simulink model "controller"  (R2024b)
settings: Solver=FixedStepDiscrete  StartTime=0.0  StopTime=30  FixedStep=0.01  RelTol=1e-3
model workspace (MAT data in the model file):
  roll = 1
undefined symbols (not defined in the file or in its folder): f
libraries: eeGeneralControl x12, slpidlib x8, dspstat3 x4, instrumentlib x4
settings Model: Creator=PC  LastModifiedBy=PC

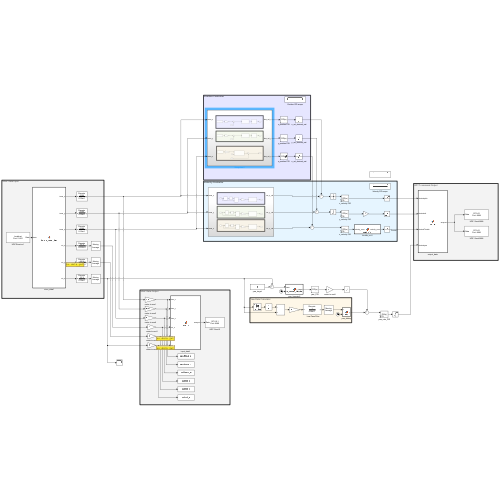
[thumbnail: Simulink's stored preview of the top-level diagram]
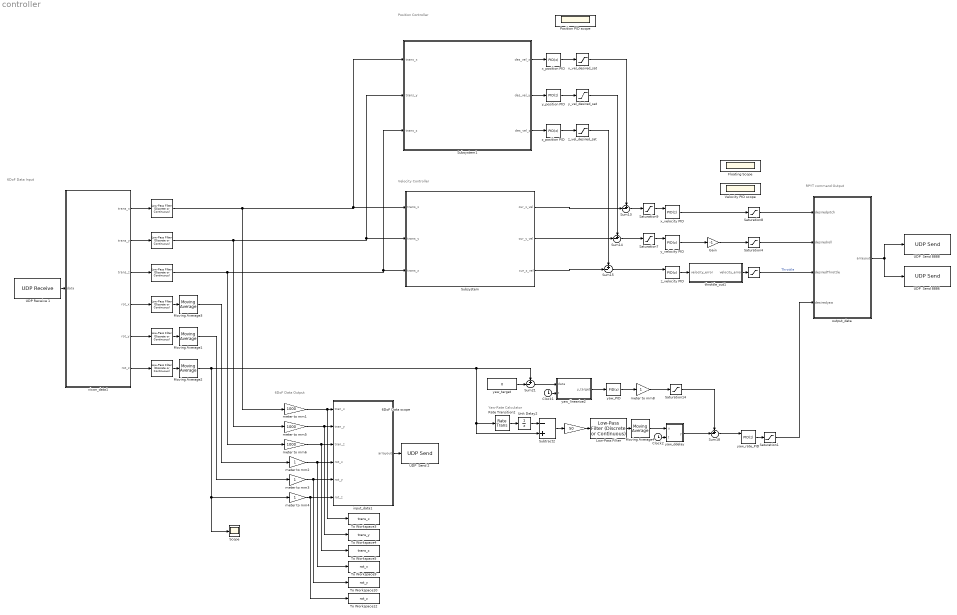
== system controller ==
  note: Velocity Controller
  note: Position Controller
  note: Yaw-Rate Calculator
  note: 6DoF Data Output
  note: 6DoF Data Input
  note: RPYT command Output
  "   " : Saturate  UpperLimit=20000  LowerLimit=0
  "    " : eeGeneralControl/Low-Pass Filter (Discrete or Continuous)  K=0.001  T=0.03  B=inf  A=-inf  init_option=Inherited from block input  x0=0  Ts=0.01
  "               " : Gain  Gain=50
  "                                       " : eeGeneralControl/Low-Pass Filter (Discrete or Continuous)  K=0.001  T=0.03  B=inf  A=-inf  init_option=Inherited from block input  x0=0  Ts=0.01
  "                                                    " : eeGeneralControl/Low-Pass Filter (Discrete or Continuous)  K=57.3  T=0.016  B=inf  A=-inf  init_option=Inherited from block input  x0=0  Ts=0.01
  "                                                      " : eeGeneralControl/Low-Pass Filter (Discrete or Continuous)  K=57.3  T=0.016  B=inf  A=-inf  init_option=Inherited from block input  x0=0  Ts=0.01
  "                                                           " : eeGeneralControl/Low-Pass Filter (Discrete or Continuous)  K=0.001  T=0.03  B=inf  A=-inf  init_option=Inherited from block input  x0=0  Ts=0.01
  "                                                                                           " : eeGeneralControl/Low-Pass Filter (Discrete or Continuous)  K=57.3  T=0.03  B=inf  A=-inf  init_option=Inherited from block input  x0=0  Ts=0.01
  "    Low-Pass Filter" : eeGeneralControl/Low-Pass Filter (Discrete or Continuous)  K=1  T=0.08  B=inf  A=-inf  init_option=Inherited from block input  x0=0  Ts=0.01
  6DoF Data scope : Scope
      settings: Floating=on
  Clock1 : Clock
  Clock2 : Clock
  Floating Scope : Scope
      settings: Floating=on
  Gain : Gain  Gain=-1
  Moving Average1 : dspstat3/Moving Average  Method=Sliding window  ForgettingFactorPort=off  SpecifyWindowLength=on  WindowLength=8  OverlapLength=7  AllowArbitraryInputLength=off  ForgettingFactor=0.9  SimulateUsing=Interpreted execution
  Moving Average2 : dspstat3/Moving Average  Method=Sliding window  ForgettingFactorPort=off  SpecifyWindowLength=on  WindowLength=15  OverlapLength=14  AllowArbitraryInputLength=off  ForgettingFactor=0.9  SimulateUsing=Interpreted execution
  Moving Average3 : dspstat3/Moving Average  Method=Sliding window  ForgettingFactorPort=off  SpecifyWindowLength=on  WindowLength=8  OverlapLength=7  AllowArbitraryInputLength=off  ForgettingFactor=0.9  SimulateUsing=Interpreted execution
  Moving Average4 : dspstat3/Moving Average  Method=Sliding window  ForgettingFactorPort=off  SpecifyWindowLength=on  WindowLength=30  OverlapLength=29  AllowArbitraryInputLength=off  ForgettingFactor=0.9  SimulateUsing=Interpreted execution
  Position PID scope : Scope
      settings: Floating=on
  Rate Transition2 : RateTransition  OutPortSampleTime=0.02
  Saturation1 : Saturate  UpperLimit=10  LowerLimit=-10
  Saturation14 : Saturate  UpperLimit=25  LowerLimit=-25
  Saturation4 : Saturate  UpperLimit=5  LowerLimit=-5
  Saturation7 : Saturate  UpperLimit=0.8  LowerLimit=-0.8
  Saturation8 : Saturate  UpperLimit=5  LowerLimit=-5
  Saturation9 : Saturate  UpperLimit=0.8  LowerLimit=-0.8
  Scope : Scope
  Subsystem : Subsystem
  Subsystem1 : Subsystem
  Subtract2 : Sum  Inputs=-+
  Sum{13..15,18,21} (5 alike) : Sum  Inputs=+-|
  To Workspace10 : ToWorkspace  VariableName=rot_y  SaveFormat=Timeseries  SampleTime=-1
  To Workspace12 : ToWorkspace  VariableName=rot_z  SaveFormat=Timeseries  SampleTime=-1
  To Workspace3 : ToWorkspace  VariableName=trans_x  SaveFormat=Timeseries  SampleTime=-1
  To Workspace4 : ToWorkspace  VariableName=trans_y  SaveFormat=Timeseries  SampleTime=-1
  To Workspace5 : ToWorkspace  VariableName=trans_z  SaveFormat=Timeseries  SampleTime=-1
  To Workspace9 : ToWorkspace  VariableName=rot_x  SaveFormat=Timeseries  SampleTime=-1
  UDP  Send 2 : instrumentlib/UDP Send  Host=127.0.0.1  Port=8889  LocalAddress=0.0.0.0  LocalPort=-1  EnablePortSharing=off  OutputDatagramPacketSize=2048  ByteOrder=big-endian  EnableBlockingMode=on  SimulateUsing=Interpreted execution
  UDP  Send 8886 : instrumentlib/UDP Send  Host=127.0.0.1  Port=8886  LocalAddress=0.0.0.0  LocalPort=-1  EnablePortSharing=off  OutputDatagramPacketSize=2048  ByteOrder=big-endian  EnableBlockingMode=on  SimulateUsing=Interpreted execution
  UDP  Send 8888 : instrumentlib/UDP Send  Host=127.0.0.1  Port=8888  LocalAddress=0.0.0.0  LocalPort=-1  EnablePortSharing=off  OutputDatagramPacketSize=2048  ByteOrder=big-endian  EnableBlockingMode=on  SimulateUsing=Interpreted execution
  UDP Receive 1 : instrumentlib/UDP Receive  LocalAddress=localhost  LocalPort=51001  EnablePortSharing=on  Host=localhost  Port=9090  GetLatestData=on  DataSize=[1024, 1]  DataType=uint8  ASCIIFormatting=%f,  Terminator=LF  CustomTerminator=10  ByteOrder=big-endian  EnableBlockingMode=on  Timeout=5  SampleTime=0.01  SimulateUsing=Interpreted execution
  Unit Delay2 : UnitDelay  SampleTime=0.01  HasFrameUpgradeWarning=on
  Velocity PID scope : Scope
      settings: Floating=on
  input_data1 : MATLAB Function  TreatAsAtomicUnit=on
  meter to mm1 : Gain  Gain=1000
  meter to mm{2..4,8} (4 alike) : Gain
  meter to mm5 : Gain  Gain=1000
  meter to mm6 : Gain  Gain=1000
  output_data : MATLAB Function  TreatAsAtomicUnit=on
  throttle_out1 : MATLAB Function  TreatAsAtomicUnit=on
  vicon_data1 : MATLAB Function  TreatAsAtomicUnit=on
  x_position PID : slpidlib/PID Controller  Controller=PID  Form=Parallel  TimeDomain=Discrete-time  UseExternalTs=off  SampleTime=-1  IntegratorMethod=Forward Euler  FilterMethod=Forward Euler  ControllerParametersSource=internal  P=2  I=0.1  UseKiTs=off  D=0.7  UseExternalDerivativeSource=off  N=50  UseFilter=on  TunerSelectOption=Transfer Function Based (PID Tuner App)  InitialConditionSource=internal  InitialConditionForIntegrator=0  InitialConditionForFilter=0  DifferentiatorICPrevScaledInput=0  ExternalReset=none  TrackingMode=off  Kt=0.1  LimitOutput=off  SatLimitsSource=internal  UpperSaturationLimit=inf  LowerSaturationLimit=-inf  LinearizeAsGain=on  AntiWindupMode=none  Kb=1  LimitIntegrator=on  UpperIntegratorSaturationLimit=0.5  LowerIntegratorSaturationLimit=-0.5  POutMin=[]  POutMax=[]  IOutMin=[]  IOutMax=[]  DOutMin=[]  DOutMax=[]  NOutMin=[]  NOutMax=[]  SumOutMin=[]  SumOutMax=[]  SaturationOutMin=[]  SaturationOutMax=[]  PParamMin=[]  PParamMax=[]  IParamMin=[]  IParamMax=[]  DParamMin=[]  DParamMax=[]  NParamMin=[]  NParamMax=[]  KbParamMin=[]  KbParamMax=[]  KtParamMin=[]  KtParamMax=[]  KbOutMin=[]  KbOutMax=[]  KtOutMin=[]  KtOutMax=[]  IntegratorOutMin=[]  IntegratorOutMax=[]  FilterOutMin=[]  FilterOutMax=[]  SumI1OutMin=[]  SumI1OutMax=[]  SumI2OutMin=[]  SumI2OutMax=[]  SumI3OutMin=[]  SumI3OutMax=[]  SumI4OutMin=[]  SumI4OutMax=[]  SumDOutMin=[]  SumDOutMax=[]  DifferentiatorOutMin=[]  DifferentiatorOutMax=[]  FilterDiffOutCoefMin=[]  FilterDiffOutCoefMax=[]  ReciprocalOutMin=[]  ReciprocalOutMax=[]  SumDenOutMin=[]  SumDenOutMax=[]  SumNumOutMin=[]  SumNumOutMax=[]  DivideOutMin=[]  DivideOutMax=[]  UdiffTsProdOutMin=[]  UdiffTsProdOutMax=[]  NTsProdOutMin=[]  NTsProdOutMax=[]  UintegralTsProdOutMin=[]  UintegralTsProdOutMax=[]  UngainTsProdOutMin=[]  UngainTsProdOutMax=[]  ClampingZeroOutDataTypeStr=Inherit: Inherit via back propagation  ClampingZeroOutMin=[]  ClampingZeroOutMax=[]  FilterDenConstantOutDataTypeStr=Inherit: Inherit via back propagation  FilterDenConstantOutMin=[]  FilterDenConstantOutMax=[]  PCopyOutDataTypeStr=Inherit: Inherit via back propagation  PCopyOutMin=[]  PCopyOutMax=[]  NCopyOutDataTypeStr=Inherit: Inherit via back propagation  NCopyOutMin=[]  NCopyOutMax=[]  IntegratorContinuousStateAttributes=''  IntegratorStateMustResolveToSignalObject=off  IntegratorRTWStateStorageClass=Auto  FilterContinuousStateAttributes=''  FilterStateMustResolveToSignalObject=off  FilterRTWStateStorageClass=Auto  ParallelPVariant=InternalParameters  IdealPVariant=Disabled  IVariant=InternalParameters  DVariant=InternalParameters  IntegratorVariant=Discrete  SatVariant=Disabled  AWVariant=Passthrough  PCopyVariant=Disabled  TRVariant=Disabled  FdbkBlocksVariant=Forward  IdealPFdbkVariant=Disabled  SatFdbkVariant=Disabled  DerivativeFilterVariant=ForwardEulerFilter  NVariant=InternalParameters  NCopyVariant=Disabled  FilterICVariant=InternalICsFilter  IntegratorICVariant=InternalICs  ExternalResetVariant=Disabled  TRSumVariant=Passthrough  SumFdbkVariant=Disabled  SumVariant=Sum_PID  TsampFilterVariant=InternalTs  TsampNgainVariant=Passthrough  TsampIntegralVariant=Disabled_SignalSpec  ExternalSaturationOutDataTypeStr=Inherit: Same as second input  DerivativeSourceVariant=ErrorSignal  PreIntVariant=InternalPreInt
  x_vel_desired_sat : Saturate  UpperLimit=1.2  LowerLimit=-1.2
  x_velocity PID : slpidlib/PID Controller  Controller=PID  Form=Parallel  TimeDomain=Discrete-time  UseExternalTs=off  SampleTime=-1  IntegratorMethod=Forward Euler  FilterMethod=Forward Euler  ControllerParametersSource=internal  P=2  I=0.2  UseKiTs=off  D=0.4  UseExternalDerivativeSource=off  N=50  UseFilter=on  TunerSelectOption=Transfer Function Based (PID Tuner App)  InitialConditionSource=internal  InitialConditionForIntegrator=0  InitialConditionForFilter=0  DifferentiatorICPrevScaledInput=0  ExternalReset=none  TrackingMode=on  Kt=1.5  LimitOutput=off  SatLimitsSource=internal  UpperSaturationLimit=inf  LowerSaturationLimit=-inf  LinearizeAsGain=on  AntiWindupMode=none  Kb=1  LimitIntegrator=on  UpperIntegratorSaturationLimit=0.3  LowerIntegratorSaturationLimit=-0.3  POutMin=[]  POutMax=[]  IOutMin=[]  IOutMax=[]  DOutMin=[]  DOutMax=[]  NOutMin=[]  NOutMax=[]  SumOutMin=[]  SumOutMax=[]  SaturationOutMin=[]  SaturationOutMax=[]  PParamMin=[]  PParamMax=[]  IParamMin=[]  IParamMax=[]  DParamMin=[]  DParamMax=[]  NParamMin=[]  NParamMax=[]  KbParamMin=[]  KbParamMax=[]  KtParamMin=[]  KtParamMax=[]  KbOutMin=[]  KbOutMax=[]  KtOutMin=[]  KtOutMax=[]  IntegratorOutMin=[]  IntegratorOutMax=[]  FilterOutMin=[]  FilterOutMax=[]  SumI1OutMin=[]  SumI1OutMax=[]  SumI2OutMin=[]  SumI2OutMax=[]  SumI3OutMin=[]  SumI3OutMax=[]  SumI4OutMin=[]  SumI4OutMax=[]  SumDOutMin=[]  SumDOutMax=[]  DifferentiatorOutMin=[]  DifferentiatorOutMax=[]  FilterDiffOutCoefMin=[]  FilterDiffOutCoefMax=[]  ReciprocalOutMin=[]  ReciprocalOutMax=[]  SumDenOutMin=[]  SumDenOutMax=[]  SumNumOutMin=[]  SumNumOutMax=[]  DivideOutMin=[]  DivideOutMax=[]  UdiffTsProdOutMin=[]  UdiffTsProdOutMax=[]  NTsProdOutMin=[]  NTsProdOutMax=[]  UintegralTsProdOutMin=[]  UintegralTsProdOutMax=[]  UngainTsProdOutMin=[]  UngainTsProdOutMax=[]  ClampingZeroOutDataTypeStr=Inherit: Inherit via back propagation  ClampingZeroOutMin=[]  ClampingZeroOutMax=[]  FilterDenConstantOutDataTypeStr=Inherit: Inherit via back propagation  FilterDenConstantOutMin=[]  FilterDenConstantOutMax=[]  PCopyOutDataTypeStr=Inherit: Inherit via back propagation  PCopyOutMin=[]  PCopyOutMax=[]  NCopyOutDataTypeStr=Inherit: Inherit via back propagation  NCopyOutMin=[]  NCopyOutMax=[]  IntegratorContinuousStateAttributes=''  IntegratorStateMustResolveToSignalObject=off  IntegratorRTWStateStorageClass=Auto  FilterContinuousStateAttributes=''  FilterStateMustResolveToSignalObject=off  FilterRTWStateStorageClass=Auto  ParallelPVariant=InternalParameters  IdealPVariant=Disabled  IVariant=InternalParameters  DVariant=InternalParameters  IntegratorVariant=Discrete  SatVariant=Disabled  AWVariant=Passthrough  PCopyVariant=Disabled  TRVariant=Enabled  FdbkBlocksVariant=Forward  IdealPFdbkVariant=Disabled  SatFdbkVariant=Disabled  DerivativeFilterVariant=ForwardEulerFilter  NVariant=InternalParameters  NCopyVariant=Disabled  FilterICVariant=InternalICsFilter  IntegratorICVariant=InternalICs  ExternalResetVariant=Disabled  TRSumVariant=TrackingMode  SumFdbkVariant=Disabled  SumVariant=Sum_PID  TsampFilterVariant=InternalTs  TsampNgainVariant=Passthrough  TsampIntegralVariant=Disabled_SignalSpec  ExternalSaturationOutDataTypeStr=Inherit: Same as second input  DerivativeSourceVariant=ErrorSignal  PreIntVariant=InternalPreInt
  y_position PID : slpidlib/PID Controller  Controller=PID  Form=Parallel  TimeDomain=Discrete-time  UseExternalTs=off  SampleTime=-1  IntegratorMethod=Forward Euler  FilterMethod=Forward Euler  ControllerParametersSource=internal  P=2  I=0.1  UseKiTs=off  D=0.7  UseExternalDerivativeSource=off  N=50  UseFilter=on  TunerSelectOption=Transfer Function Based (PID Tuner App)  InitialConditionSource=internal  InitialConditionForIntegrator=0  InitialConditionForFilter=0  DifferentiatorICPrevScaledInput=0  ExternalReset=none  TrackingMode=off  Kt=0.1  LimitOutput=off  SatLimitsSource=internal  UpperSaturationLimit=inf  LowerSaturationLimit=-inf  LinearizeAsGain=on  AntiWindupMode=none  Kb=1  LimitIntegrator=on  UpperIntegratorSaturationLimit=0.5  LowerIntegratorSaturationLimit=-0.5  POutMin=[]  POutMax=[]  IOutMin=[]  IOutMax=[]  DOutMin=[]  DOutMax=[]  NOutMin=[]  NOutMax=[]  SumOutMin=[]  SumOutMax=[]  SaturationOutMin=[]  SaturationOutMax=[]  PParamMin=[]  PParamMax=[]  IParamMin=[]  IParamMax=[]  DParamMin=[]  DParamMax=[]  NParamMin=[]  NParamMax=[]  KbParamMin=[]  KbParamMax=[]  KtParamMin=[]  KtParamMax=[]  KbOutMin=[]  KbOutMax=[]  KtOutMin=[]  KtOutMax=[]  IntegratorOutMin=[]  IntegratorOutMax=[]  FilterOutMin=[]  FilterOutMax=[]  SumI1OutMin=[]  SumI1OutMax=[]  SumI2OutMin=[]  SumI2OutMax=[]  SumI3OutMin=[]  SumI3OutMax=[]  SumI4OutMin=[]  SumI4OutMax=[]  SumDOutMin=[]  SumDOutMax=[]  DifferentiatorOutMin=[]  DifferentiatorOutMax=[]  FilterDiffOutCoefMin=[]  FilterDiffOutCoefMax=[]  ReciprocalOutMin=[]  ReciprocalOutMax=[]  SumDenOutMin=[]  SumDenOutMax=[]  SumNumOutMin=[]  SumNumOutMax=[]  DivideOutMin=[]  DivideOutMax=[]  UdiffTsProdOutMin=[]  UdiffTsProdOutMax=[]  NTsProdOutMin=[]  NTsProdOutMax=[]  UintegralTsProdOutMin=[]  UintegralTsProdOutMax=[]  UngainTsProdOutMin=[]  UngainTsProdOutMax=[]  ClampingZeroOutDataTypeStr=Inherit: Inherit via back propagation  ClampingZeroOutMin=[]  ClampingZeroOutMax=[]  FilterDenConstantOutDataTypeStr=Inherit: Inherit via back propagation  FilterDenConstantOutMin=[]  FilterDenConstantOutMax=[]  PCopyOutDataTypeStr=Inherit: Inherit via back propagation  PCopyOutMin=[]  PCopyOutMax=[]  NCopyOutDataTypeStr=Inherit: Inherit via back propagation  NCopyOutMin=[]  NCopyOutMax=[]  IntegratorContinuousStateAttributes=''  IntegratorStateMustResolveToSignalObject=off  IntegratorRTWStateStorageClass=Auto  FilterContinuousStateAttributes=''  FilterStateMustResolveToSignalObject=off  FilterRTWStateStorageClass=Auto  ParallelPVariant=InternalParameters  IdealPVariant=Disabled  IVariant=InternalParameters  DVariant=InternalParameters  IntegratorVariant=Discrete  SatVariant=Disabled  AWVariant=Passthrough  PCopyVariant=Disabled  TRVariant=Disabled  FdbkBlocksVariant=Forward  IdealPFdbkVariant=Disabled  SatFdbkVariant=Disabled  DerivativeFilterVariant=ForwardEulerFilter  NVariant=InternalParameters  NCopyVariant=Disabled  FilterICVariant=InternalICsFilter  IntegratorICVariant=InternalICs  ExternalResetVariant=Disabled  TRSumVariant=Passthrough  SumFdbkVariant=Disabled  SumVariant=Sum_PID  TsampFilterVariant=InternalTs  TsampNgainVariant=Passthrough  TsampIntegralVariant=Disabled_SignalSpec  ExternalSaturationOutDataTypeStr=Inherit: Same as second input  DerivativeSourceVariant=ErrorSignal  PreIntVariant=InternalPreInt
  y_vel_desired_sat : Saturate  UpperLimit=1.2  LowerLimit=-1.2
  y_velocity PID : slpidlib/PID Controller  Controller=PID  Form=Parallel  TimeDomain=Discrete-time  UseExternalTs=off  SampleTime=-1  IntegratorMethod=Forward Euler  FilterMethod=Forward Euler  ControllerParametersSource=internal  P=3.2  I=0.06  UseKiTs=off  D=0.25  UseExternalDerivativeSource=off  N=50  UseFilter=on  TunerSelectOption=Transfer Function Based (PID Tuner App)  InitialConditionSource=internal  InitialConditionForIntegrator=0  InitialConditionForFilter=0  DifferentiatorICPrevScaledInput=0  ExternalReset=none  TrackingMode=on  Kt=1.7  LimitOutput=off  SatLimitsSource=internal  UpperSaturationLimit=inf  LowerSaturationLimit=-inf  LinearizeAsGain=on  AntiWindupMode=none  Kb=1  LimitIntegrator=on  UpperIntegratorSaturationLimit=0.3  LowerIntegratorSaturationLimit=-0.3  POutMin=[]  POutMax=[]  IOutMin=[]  IOutMax=[]  DOutMin=[]  DOutMax=[]  NOutMin=[]  NOutMax=[]  SumOutMin=[]  SumOutMax=[]  SaturationOutMin=[]  SaturationOutMax=[]  PParamMin=[]  PParamMax=[]  IParamMin=[]  IParamMax=[]  DParamMin=[]  DParamMax=[]  NParamMin=[]  NParamMax=[]  KbParamMin=[]  KbParamMax=[]  KtParamMin=[]  KtParamMax=[]  KbOutMin=[]  KbOutMax=[]  KtOutMin=[]  KtOutMax=[]  IntegratorOutMin=[]  IntegratorOutMax=[]  FilterOutMin=[]  FilterOutMax=[]  SumI1OutMin=[]  SumI1OutMax=[]  SumI2OutMin=[]  SumI2OutMax=[]  SumI3OutMin=[]  SumI3OutMax=[]  SumI4OutMin=[]  SumI4OutMax=[]  SumDOutMin=[]  SumDOutMax=[]  DifferentiatorOutMin=[]  DifferentiatorOutMax=[]  FilterDiffOutCoefMin=[]  FilterDiffOutCoefMax=[]  ReciprocalOutMin=[]  ReciprocalOutMax=[]  SumDenOutMin=[]  SumDenOutMax=[]  SumNumOutMin=[]  SumNumOutMax=[]  DivideOutMin=[]  DivideOutMax=[]  UdiffTsProdOutMin=[]  UdiffTsProdOutMax=[]  NTsProdOutMin=[]  NTsProdOutMax=[]  UintegralTsProdOutMin=[]  UintegralTsProdOutMax=[]  UngainTsProdOutMin=[]  UngainTsProdOutMax=[]  ClampingZeroOutDataTypeStr=Inherit: Inherit via back propagation  ClampingZeroOutMin=[]  ClampingZeroOutMax=[]  FilterDenConstantOutDataTypeStr=Inherit: Inherit via back propagation  FilterDenConstantOutMin=[]  FilterDenConstantOutMax=[]  PCopyOutDataTypeStr=Inherit: Inherit via back propagation  PCopyOutMin=[]  PCopyOutMax=[]  NCopyOutDataTypeStr=Inherit: Inherit via back propagation  NCopyOutMin=[]  NCopyOutMax=[]  IntegratorContinuousStateAttributes=''  IntegratorStateMustResolveToSignalObject=off  IntegratorRTWStateStorageClass=Auto  FilterContinuousStateAttributes=''  FilterStateMustResolveToSignalObject=off  FilterRTWStateStorageClass=Auto  ParallelPVariant=InternalParameters  IdealPVariant=Disabled  IVariant=InternalParameters  DVariant=InternalParameters  IntegratorVariant=Discrete  SatVariant=Disabled  AWVariant=Passthrough  PCopyVariant=Disabled  TRVariant=Enabled  FdbkBlocksVariant=Forward  IdealPFdbkVariant=Disabled  SatFdbkVariant=Disabled  DerivativeFilterVariant=ForwardEulerFilter  NVariant=InternalParameters  NCopyVariant=Disabled  FilterICVariant=InternalICsFilter  IntegratorICVariant=InternalICs  ExternalResetVariant=Disabled  TRSumVariant=TrackingMode  SumFdbkVariant=Disabled  SumVariant=Sum_PID  TsampFilterVariant=InternalTs  TsampNgainVariant=Passthrough  TsampIntegralVariant=Disabled_SignalSpec  ExternalSaturationOutDataTypeStr=Inherit: Same as second input  DerivativeSourceVariant=ErrorSignal  PreIntVariant=InternalPreInt
  yaw_PID : slpidlib/PID Controller  Controller=PID  Form=Parallel  TimeDomain=Discrete-time  UseExternalTs=off  SampleTime=-1  IntegratorMethod=Forward Euler  FilterMethod=Forward Euler  ControllerParametersSource=internal  P=0.3  I=0.05  UseKiTs=off  D=0  UseExternalDerivativeSource=off  N=50  UseFilter=on  TunerSelectOption=Transfer Function Based (PID Tuner App)  InitialConditionSource=internal  InitialConditionForIntegrator=0  InitialConditionForFilter=0  DifferentiatorICPrevScaledInput=0  ExternalReset=none  TrackingMode=off  Kt=4  LimitOutput=off  SatLimitsSource=internal  UpperSaturationLimit=inf  LowerSaturationLimit=-inf  LinearizeAsGain=on  AntiWindupMode=none  Kb=1  LimitIntegrator=on  UpperIntegratorSaturationLimit=2  LowerIntegratorSaturationLimit=-2  POutMin=[]  POutMax=[]  IOutMin=[]  IOutMax=[]  DOutMin=[]  DOutMax=[]  NOutMin=[]  NOutMax=[]  SumOutMin=[]  SumOutMax=[]  SaturationOutMin=[]  SaturationOutMax=[]  PParamMin=[]  PParamMax=[]  IParamMin=[]  IParamMax=[]  DParamMin=[]  DParamMax=[]  NParamMin=[]  NParamMax=[]  KbParamMin=[]  KbParamMax=[]  KtParamMin=[]  KtParamMax=[]  KbOutMin=[]  KbOutMax=[]  KtOutMin=[]  KtOutMax=[]  IntegratorOutMin=[]  IntegratorOutMax=[]  FilterOutMin=[]  FilterOutMax=[]  SumI1OutMin=[]  SumI1OutMax=[]  SumI2OutMin=[]  SumI2OutMax=[]  SumI3OutMin=[]  SumI3OutMax=[]  SumI4OutMin=[]  SumI4OutMax=[]  SumDOutMin=[]  SumDOutMax=[]  DifferentiatorOutMin=[]  DifferentiatorOutMax=[]  FilterDiffOutCoefMin=[]  FilterDiffOutCoefMax=[]  ReciprocalOutMin=[]  ReciprocalOutMax=[]  SumDenOutMin=[]  SumDenOutMax=[]  SumNumOutMin=[]  SumNumOutMax=[]  DivideOutMin=[]  DivideOutMax=[]  UdiffTsProdOutMin=[]  UdiffTsProdOutMax=[]  NTsProdOutMin=[]  NTsProdOutMax=[]  UintegralTsProdOutMin=[]  UintegralTsProdOutMax=[]  UngainTsProdOutMin=[]  UngainTsProdOutMax=[]  ClampingZeroOutDataTypeStr=Inherit: Inherit via back propagation  ClampingZeroOutMin=[]  ClampingZeroOutMax=[]  FilterDenConstantOutDataTypeStr=Inherit: Inherit via back propagation  FilterDenConstantOutMin=[]  FilterDenConstantOutMax=[]  PCopyOutDataTypeStr=Inherit: Inherit via back propagation  PCopyOutMin=[]  PCopyOutMax=[]  NCopyOutDataTypeStr=Inherit: Inherit via back propagation  NCopyOutMin=[]  NCopyOutMax=[]  IntegratorContinuousStateAttributes=''  IntegratorStateMustResolveToSignalObject=off  IntegratorRTWStateStorageClass=Auto  FilterContinuousStateAttributes=''  FilterStateMustResolveToSignalObject=off  FilterRTWStateStorageClass=Auto  ParallelPVariant=InternalParameters  IdealPVariant=Disabled  IVariant=InternalParameters  DVariant=InternalParameters  IntegratorVariant=Discrete  SatVariant=Disabled  AWVariant=Passthrough  PCopyVariant=Disabled  TRVariant=Disabled  FdbkBlocksVariant=Forward  IdealPFdbkVariant=Disabled  SatFdbkVariant=Disabled  DerivativeFilterVariant=ForwardEulerFilter  NVariant=InternalParameters  NCopyVariant=Disabled  FilterICVariant=InternalICsFilter  IntegratorICVariant=InternalICs  ExternalResetVariant=Disabled  TRSumVariant=Passthrough  SumFdbkVariant=Disabled  SumVariant=Sum_PID  TsampFilterVariant=InternalTs  TsampNgainVariant=Passthrough  TsampIntegralVariant=Disabled_SignalSpec  ExternalSaturationOutDataTypeStr=Inherit: Same as second input  DerivativeSourceVariant=ErrorSignal  PreIntVariant=InternalPreInt
  yaw_ddelay : MATLAB Function  TreatAsAtomicUnit=on
  yaw_linearize2 : MATLAB Function  TreatAsAtomicUnit=on
  yaw_rate_PID : slpidlib/PID Controller  Controller=PID  Form=Parallel  TimeDomain=Discrete-time  UseExternalTs=off  SampleTime=-1  IntegratorMethod=Forward Euler  FilterMethod=Forward Euler  ControllerParametersSource=internal  P=1  I=0  UseKiTs=off  D=0  UseExternalDerivativeSource=off  N=50  UseFilter=on  TunerSelectOption=Transfer Function Based (PID Tuner App)  InitialConditionSource=internal  InitialConditionForIntegrator=0  InitialConditionForFilter=0  DifferentiatorICPrevScaledInput=0  ExternalReset=none  TrackingMode=on  Kt=2  LimitOutput=off  SatLimitsSource=internal  UpperSaturationLimit=inf  LowerSaturationLimit=-inf  LinearizeAsGain=on  AntiWindupMode=none  Kb=1  LimitIntegrator=on  UpperIntegratorSaturationLimit=2  LowerIntegratorSaturationLimit=-2  POutMin=[]  POutMax=[]  IOutMin=[]  IOutMax=[]  DOutMin=[]  DOutMax=[]  NOutMin=[]  NOutMax=[]  SumOutMin=[]  SumOutMax=[]  SaturationOutMin=[]  SaturationOutMax=[]  PParamMin=[]  PParamMax=[]  IParamMin=[]  IParamMax=[]  DParamMin=[]  DParamMax=[]  NParamMin=[]  NParamMax=[]  KbParamMin=[]  KbParamMax=[]  KtParamMin=[]  KtParamMax=[]  KbOutMin=[]  KbOutMax=[]  KtOutMin=[]  KtOutMax=[]  IntegratorOutMin=[]  IntegratorOutMax=[]  FilterOutMin=[]  FilterOutMax=[]  SumI1OutMin=[]  SumI1OutMax=[]  SumI2OutMin=[]  SumI2OutMax=[]  SumI3OutMin=[]  SumI3OutMax=[]  SumI4OutMin=[]  SumI4OutMax=[]  SumDOutMin=[]  SumDOutMax=[]  DifferentiatorOutMin=[]  DifferentiatorOutMax=[]  FilterDiffOutCoefMin=[]  FilterDiffOutCoefMax=[]  ReciprocalOutMin=[]  ReciprocalOutMax=[]  SumDenOutMin=[]  SumDenOutMax=[]  SumNumOutMin=[]  SumNumOutMax=[]  DivideOutMin=[]  DivideOutMax=[]  UdiffTsProdOutMin=[]  UdiffTsProdOutMax=[]  NTsProdOutMin=[]  NTsProdOutMax=[]  UintegralTsProdOutMin=[]  UintegralTsProdOutMax=[]  UngainTsProdOutMin=[]  UngainTsProdOutMax=[]  ClampingZeroOutDataTypeStr=Inherit: Inherit via back propagation  ClampingZeroOutMin=[]  ClampingZeroOutMax=[]  FilterDenConstantOutDataTypeStr=Inherit: Inherit via back propagation  FilterDenConstantOutMin=[]  FilterDenConstantOutMax=[]  PCopyOutDataTypeStr=Inherit: Inherit via back propagation  PCopyOutMin=[]  PCopyOutMax=[]  NCopyOutDataTypeStr=Inherit: Inherit via back propagation  NCopyOutMin=[]  NCopyOutMax=[]  IntegratorContinuousStateAttributes=''  IntegratorStateMustResolveToSignalObject=off  IntegratorRTWStateStorageClass=Auto  FilterContinuousStateAttributes=''  FilterStateMustResolveToSignalObject=off  FilterRTWStateStorageClass=Auto  ParallelPVariant=InternalParameters  IdealPVariant=Disabled  IVariant=InternalParameters  DVariant=InternalParameters  IntegratorVariant=Discrete  SatVariant=Disabled  AWVariant=Passthrough  PCopyVariant=Disabled  TRVariant=Enabled  FdbkBlocksVariant=Forward  IdealPFdbkVariant=Disabled  SatFdbkVariant=Disabled  DerivativeFilterVariant=ForwardEulerFilter  NVariant=InternalParameters  NCopyVariant=Disabled  FilterICVariant=InternalICsFilter  IntegratorICVariant=InternalICs  ExternalResetVariant=Disabled  TRSumVariant=TrackingMode  SumFdbkVariant=Disabled  SumVariant=Sum_PID  TsampFilterVariant=InternalTs  TsampNgainVariant=Passthrough  TsampIntegralVariant=Disabled_SignalSpec  ExternalSaturationOutDataTypeStr=Inherit: Same as second input  DerivativeSourceVariant=ErrorSignal  PreIntVariant=InternalPreInt
  yaw_target : Constant  Value=0
  z_position PID : slpidlib/PID Controller  Controller=PID  Form=Parallel  TimeDomain=Discrete-time  UseExternalTs=off  SampleTime=-1  IntegratorMethod=Forward Euler  FilterMethod=Forward Euler  ControllerParametersSource=internal  P=1  I=0.5  UseKiTs=off  D=0  UseExternalDerivativeSource=off  N=50  UseFilter=on  TunerSelectOption=Frequency Response Based  InitialConditionSource=internal  InitialConditionForIntegrator=0  InitialConditionForFilter=0  DifferentiatorICPrevScaledInput=0  ExternalReset=none  TrackingMode=off  Kt=1  LimitOutput=on  SatLimitsSource=internal  UpperSaturationLimit=3  LowerSaturationLimit=-3  LinearizeAsGain=on  AntiWindupMode=clamping  Kb=1  LimitIntegrator=on  UpperIntegratorSaturationLimit=0.5  LowerIntegratorSaturationLimit=-0.5  POutMin=[]  POutMax=[]  IOutMin=[]  IOutMax=[]  DOutMin=[]  DOutMax=[]  NOutMin=[]  NOutMax=[]  SumOutMin=[]  SumOutMax=[]  SaturationOutMin=[]  SaturationOutMax=[]  PParamMin=[]  PParamMax=[]  IParamMin=[]  IParamMax=[]  DParamMin=[]  DParamMax=[]  NParamMin=[]  NParamMax=[]  KbParamMin=[]  KbParamMax=[]  KtParamMin=[]  KtParamMax=[]  KbOutMin=[]  KbOutMax=[]  KtOutMin=[]  KtOutMax=[]  IntegratorOutMin=[]  IntegratorOutMax=[]  FilterOutMin=[]  FilterOutMax=[]  SumI1OutMin=[]  SumI1OutMax=[]  SumI2OutMin=[]  SumI2OutMax=[]  SumI3OutMin=[]  SumI3OutMax=[]  SumI4OutMin=[]  SumI4OutMax=[]  SumDOutMin=[]  SumDOutMax=[]  DifferentiatorOutMin=[]  DifferentiatorOutMax=[]  FilterDiffOutCoefMin=[]  FilterDiffOutCoefMax=[]  ReciprocalOutMin=[]  ReciprocalOutMax=[]  SumDenOutMin=[]  SumDenOutMax=[]  SumNumOutMin=[]  SumNumOutMax=[]  DivideOutMin=[]  DivideOutMax=[]  UdiffTsProdOutMin=[]  UdiffTsProdOutMax=[]  NTsProdOutMin=[]  NTsProdOutMax=[]  UintegralTsProdOutMin=[]  UintegralTsProdOutMax=[]  UngainTsProdOutMin=[]  UngainTsProdOutMax=[]  ClampingZeroOutDataTypeStr=Inherit: Inherit via back propagation  ClampingZeroOutMin=[]  ClampingZeroOutMax=[]  FilterDenConstantOutDataTypeStr=Inherit: Inherit via back propagation  FilterDenConstantOutMin=[]  FilterDenConstantOutMax=[]  PCopyOutDataTypeStr=Inherit: Inherit via back propagation  PCopyOutMin=[]  PCopyOutMax=[]  NCopyOutDataTypeStr=Inherit: Inherit via back propagation  NCopyOutMin=[]  NCopyOutMax=[]  IntegratorContinuousStateAttributes=''  IntegratorStateMustResolveToSignalObject=off  IntegratorRTWStateStorageClass=Auto  FilterContinuousStateAttributes=''  FilterStateMustResolveToSignalObject=off  FilterRTWStateStorageClass=Auto  ParallelPVariant=InternalParameters  IdealPVariant=Disabled  IVariant=InternalParameters  DVariant=InternalParameters  IntegratorVariant=Discrete  SatVariant=Enabled  AWVariant=DiscClampingParallel  PCopyVariant=Disabled  TRVariant=Disabled  FdbkBlocksVariant=Forward  IdealPFdbkVariant=Disabled  SatFdbkVariant=Disabled  DerivativeFilterVariant=ForwardEulerFilter  NVariant=InternalParameters  NCopyVariant=Disabled  FilterICVariant=InternalICsFilter  IntegratorICVariant=InternalICs  ExternalResetVariant=Disabled  TRSumVariant=Passthrough  SumFdbkVariant=Disabled  SumVariant=Sum_PID  TsampFilterVariant=InternalTs  TsampNgainVariant=Passthrough  TsampIntegralVariant=Disabled_SignalSpec  ExternalSaturationOutDataTypeStr=Inherit: Same as second input  DerivativeSourceVariant=ErrorSignal  PreIntVariant=InternalPreInt
  z_vel_desired_sat : Saturate  UpperLimit=2  LowerLimit=-2
  z_velocity PID : slpidlib/PID Controller  Controller=PID  Form=Parallel  TimeDomain=Discrete-time  UseExternalTs=off  SampleTime=-1  IntegratorMethod=Forward Euler  FilterMethod=Forward Euler  ControllerParametersSource=internal  P=25  I=15  UseKiTs=off  D=0  UseExternalDerivativeSource=off  N=50  UseFilter=on  TunerSelectOption=Transfer Function Based (PID Tuner App)  InitialConditionSource=internal  InitialConditionForIntegrator=0  InitialConditionForFilter=0  DifferentiatorICPrevScaledInput=0  ExternalReset=none  TrackingMode=on  Kt=0.2  LimitOutput=off  SatLimitsSource=internal  UpperSaturationLimit=inf  LowerSaturationLimit=-inf  LinearizeAsGain=on  AntiWindupMode=none  Kb=1  LimitIntegrator=off  UpperIntegratorSaturationLimit=inf  LowerIntegratorSaturationLimit=-inf  POutMin=[]  POutMax=[]  IOutMin=[]  IOutMax=[]  DOutMin=[]  DOutMax=[]  NOutMin=[]  NOutMax=[]  SumOutMin=[]  SumOutMax=[]  SaturationOutMin=[]  SaturationOutMax=[]  PParamMin=[]  PParamMax=[]  IParamMin=[]  IParamMax=[]  DParamMin=[]  DParamMax=[]  NParamMin=[]  NParamMax=[]  KbParamMin=[]  KbParamMax=[]  KtParamMin=[]  KtParamMax=[]  KbOutMin=[]  KbOutMax=[]  KtOutMin=[]  KtOutMax=[]  IntegratorOutMin=[]  IntegratorOutMax=[]  FilterOutMin=[]  FilterOutMax=[]  SumI1OutMin=[]  SumI1OutMax=[]  SumI2OutMin=[]  SumI2OutMax=[]  SumI3OutMin=[]  SumI3OutMax=[]  SumI4OutMin=[]  SumI4OutMax=[]  SumDOutMin=[]  SumDOutMax=[]  DifferentiatorOutMin=[]  DifferentiatorOutMax=[]  FilterDiffOutCoefMin=[]  FilterDiffOutCoefMax=[]  ReciprocalOutMin=[]  ReciprocalOutMax=[]  SumDenOutMin=[]  SumDenOutMax=[]  SumNumOutMin=[]  SumNumOutMax=[]  DivideOutMin=[]  DivideOutMax=[]  UdiffTsProdOutMin=[]  UdiffTsProdOutMax=[]  NTsProdOutMin=[]  NTsProdOutMax=[]  UintegralTsProdOutMin=[]  UintegralTsProdOutMax=[]  UngainTsProdOutMin=[]  UngainTsProdOutMax=[]  ClampingZeroOutDataTypeStr=Inherit: Inherit via back propagation  ClampingZeroOutMin=[]  ClampingZeroOutMax=[]  FilterDenConstantOutDataTypeStr=Inherit: Inherit via back propagation  FilterDenConstantOutMin=[]  FilterDenConstantOutMax=[]  PCopyOutDataTypeStr=Inherit: Inherit via back propagation  PCopyOutMin=[]  PCopyOutMax=[]  NCopyOutDataTypeStr=Inherit: Inherit via back propagation  NCopyOutMin=[]  NCopyOutMax=[]  IntegratorContinuousStateAttributes=''  IntegratorStateMustResolveToSignalObject=off  IntegratorRTWStateStorageClass=Auto  FilterContinuousStateAttributes=''  FilterStateMustResolveToSignalObject=off  FilterRTWStateStorageClass=Auto  ParallelPVariant=InternalParameters  IdealPVariant=Disabled  IVariant=InternalParameters  DVariant=InternalParameters  IntegratorVariant=Discrete  SatVariant=Disabled  AWVariant=Passthrough  PCopyVariant=Disabled  TRVariant=Enabled  FdbkBlocksVariant=Forward  IdealPFdbkVariant=Disabled  SatFdbkVariant=Disabled  DerivativeFilterVariant=ForwardEulerFilter  NVariant=InternalParameters  NCopyVariant=Disabled  FilterICVariant=InternalICsFilter  IntegratorICVariant=InternalICs  ExternalResetVariant=Disabled  TRSumVariant=TrackingMode  SumFdbkVariant=Disabled  SumVariant=Sum_PID  TsampFilterVariant=InternalTs  TsampNgainVariant=Passthrough  TsampIntegralVariant=Disabled_SignalSpec  ExternalSaturationOutDataTypeStr=Inherit: Same as second input  DerivativeSourceVariant=ErrorSignal  PreIntVariant=InternalPreInt
  wires:
  output_data/1(arrayout) -> UDP  Send 8886/1, UDP  Send 8888/1
  Moving Average3/1 -> meter to mm2/1
  "                                                    "/1 -> Moving Average3/1
  Moving Average1/1 -> meter to mm3/1
  x_velocity PID/1 -> Saturation8/1
  "                                                                                           "/1 -> Moving Average2/1
  "                                                      "/1 -> Moving Average1/1
  y_velocity PID/1 -> Gain/1
  z_position PID/1 -> z_vel_desired_sat/1
  vicon_data1/1(trans_x) -> "                                       "/1
  meter to mm5/1 -> To Workspace4/1, input_data1/2(tran_y)
  Saturation7/1 -> y_velocity PID/1
  meter to mm6/1 -> To Workspace5/1, input_data1/3(tran_z)
  meter to mm4/1 -> To Workspace12/1, input_data1/6(rot_z)
  "    "/1 -> Subsystem1/2(trans_y), Subsystem/2(trans_y), meter to mm5/1
  vicon_data1/3(trans_z) -> "                                                           "/1
  Subsystem/1(cur_x_vel) -> Sum13/2
  Saturation9/1 -> x_velocity PID/1
  Sum15/1 -> z_velocity PID/1
  vicon_data1/5(rot_y) -> "                                                      "/1
  z_velocity PID/1 -> throttle_out1/1("velocity_error ")
  vicon_data1/6(rot_z) -> "                                                                                           "/1
  Subsystem/3(cur_z_vel) -> Sum15/2
  z_vel_desired_sat/1 -> Sum15/1
  Sum14/1 -> Saturation7/1
  "                                                           "/1 -> meter to mm6/1, Subsystem1/3(trans_z), Subsystem/3(trans_z)
  input_data1/1(arrayout) -> UDP  Send 2/1
  Sum13/1 -> Saturation9/1
  UDP Receive 1/1 -> vicon_data1/1(data)
  Subsystem1/2(des_vel_y) -> y_position PID/1
  meter to mm3/1 -> To Workspace10/1, input_data1/5(rot_y)
  vicon_data1/2(trans_y) -> "    "/1
  throttle_out1/1(velocity_error) -> "   "/1
  Subsystem1/1(des_vel_x) -> x_position PID/1
  Subsystem/2(cur_y_vel) -> Sum14/2
  vicon_data1/4(rot_x) -> "                                                    "/1
  "                                       "/1 -> Subsystem1/1(trans_x), Subsystem/1(trans_x), meter to mm1/1
  y_position PID/1 -> y_vel_desired_sat/1
  y_vel_desired_sat/1 -> Sum14/1
  Subsystem1/3(des_vel_z) -> z_position PID/1
  meter to mm2/1 -> To Workspace9/1, input_data1/4(rot_x)
  x_vel_desired_sat/1 -> Sum13/1
  x_position PID/1 -> x_vel_desired_sat/1
  meter to mm1/1 -> To Workspace3/1, input_data1/1(tran_x)
  "   "/1 -> output_data/3(desiredThrottle)  "Throttle"
  Saturation8/1 -> output_data/1(desiredpitch)
  Saturation4/1 -> output_data/2(desiredroll)
  yaw_target/1 -> Sum21/2
  Clock1/1 -> yaw_linearize2/2(t)
  Sum21/1 -> yaw_linearize2/1(data)
  yaw_linearize2/1(y_target) -> yaw_PID/1
  Subtract2/1 -> "               "/1
  Rate Transition2/1 -> Unit Delay2/1
  "               "/1 -> "    Low-Pass Filter"/1
  Moving Average2/1 -> Subtract2/2, Rate Transition2/1, Sum21/1, meter to mm4/1, Scope/1
  Unit Delay2/1 -> Subtract2/1
  "    Low-Pass Filter"/1 -> Moving Average4/1
  Saturation14/1 -> Sum18/1
  yaw_rate_PID/1 -> Saturation1/1
  yaw_PID/1 -> meter to mm8/1
  Moving Average4/1 -> yaw_ddelay/1(u)
  yaw_ddelay/1(y) -> Sum18/2
  Clock2/1 -> yaw_ddelay/2(t)
  Gain/1 -> Saturation4/1
  Saturation1/1 -> output_data/4(desiredyaw)
  Sum18/1 -> yaw_rate_PID/1
  meter to mm8/1 -> Saturation14/1

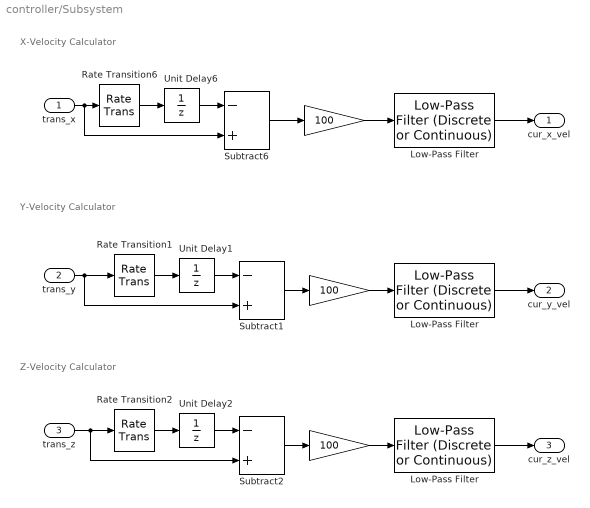
== system controller/Subsystem ==
  note: Y-Velocity Calculator
  note: X-Velocity Calculator
  note: Z-Velocity Calculator
  trans_x : Inport
  trans_y : Inport  Port=2
  trans_z : Inport  Port=3
  "  " : Gain  Gain=100
  "   " : Gain  Gain=100
  "     " : Gain  Gain=100
  "   Low-Pass Filter" : eeGeneralControl/Low-Pass Filter (Discrete or Continuous)  K=1  T=0.05  B=inf  A=-inf  init_option=Inherited from block input  x0=0  Ts=0.01
  "  Low-Pass Filter" : eeGeneralControl/Low-Pass Filter (Discrete or Continuous)  K=1  T=0.06  B=inf  A=-inf  init_option=Inherited from block input  x0=0  Ts=0.01
  "  Low-Pass Filter  " : eeGeneralControl/Low-Pass Filter (Discrete or Continuous)  K=1  T=0.06  B=inf  A=-inf  init_option=Inherited from block input  x0=0  Ts=0.01
  Rate Transition1 : RateTransition  OutPortSampleTime=0.01
  Rate Transition2 : RateTransition  OutPortSampleTime=0.01
  Rate Transition6 : RateTransition  OutPortSampleTime=0.01
  Subtract1 : Sum  Inputs=-+
  Subtract2 : Sum  Inputs=-+
  Subtract6 : Sum  Inputs=-+
  Unit Delay1 : UnitDelay  SampleTime=0.01  HasFrameUpgradeWarning=on
  Unit Delay2 : UnitDelay  SampleTime=0.01  HasFrameUpgradeWarning=on
  Unit Delay6 : UnitDelay  SampleTime=0.01  HasFrameUpgradeWarning=on
  cur_x_vel : Outport
  cur_y_vel : Outport  Port=2
  cur_z_vel : Outport  Port=3
  wires:
  "  "/1 -> "  Low-Pass Filter"/1
  Subtract6/1 -> "  "/1
  trans_x/1 -> Subtract6/2, Rate Transition6/1
  "  Low-Pass Filter"/1 -> cur_x_vel/1
  Rate Transition6/1 -> Unit Delay6/1
  Unit Delay6/1 -> Subtract6/1
  Subtract1/1 -> "   "/1
  "   "/1 -> "  Low-Pass Filter  "/1
  Unit Delay1/1 -> Subtract1/1
  Rate Transition1/1 -> Unit Delay1/1
  "     "/1 -> "   Low-Pass Filter"/1
  Unit Delay2/1 -> Subtract2/1
  Subtract2/1 -> "     "/1
  Rate Transition2/1 -> Unit Delay2/1
  trans_y/1 -> Subtract1/2, Rate Transition1/1
  trans_z/1 -> Subtract2/2, Rate Transition2/1
  "  Low-Pass Filter  "/1 -> cur_y_vel/1
  "   Low-Pass Filter"/1 -> cur_z_vel/1

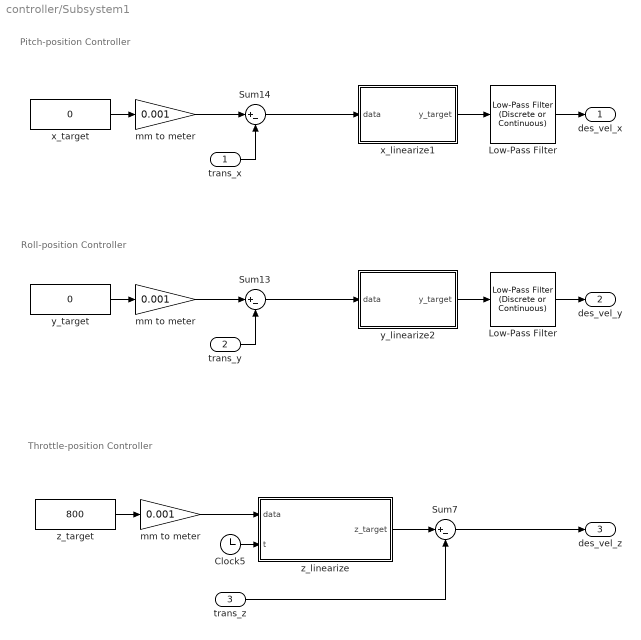
== system controller/Subsystem1 ==
  note: Pitch-position Controller
  note: Roll-position Controller
  note: Throttle-position Controller
  trans_x : Inport
  trans_y : Inport  Port=2
  trans_z : Inport  Port=3
  " mm to meter" : Gain  Gain=0.001
  " mm to meter " : Gain  Gain=0.001
  Clock5 : Clock
  Low-Pass Filter : eeGeneralControl/Low-Pass Filter (Discrete or Continuous)  K=1  T=0.08  B=inf  A=-inf  init_option=Inherited from block input  x0=0  Ts=0.01
  "Low-Pass Filter " : eeGeneralControl/Low-Pass Filter (Discrete or Continuous)  K=1  T=0.08  B=inf  A=-inf  init_option=Inherited from block input  x0=0  Ts=0.01
  Sum13 : Sum  Inputs=|+-
  Sum14 : Sum  Inputs=|+-
  Sum7 : Sum  Inputs=|+-
  mm to meter : Gain  Gain=0.001
  x_linearize1 : MATLAB Function  TreatAsAtomicUnit=on
  x_target : Constant  Value=0
  y_linearize2 : MATLAB Function  TreatAsAtomicUnit=on
  y_target : Constant  Value=0
  z_linearize : MATLAB Function  TreatAsAtomicUnit=on
  z_target : Constant  Value=800
  des_vel_x : Outport
  des_vel_y : Outport  Port=2
  des_vel_z : Outport  Port=3
  wires:
  y_target/1 -> mm to meter/1
  Low-Pass Filter/1 -> des_vel_x/1
  y_linearize2/1(y_target) -> "Low-Pass Filter "/1
  mm to meter/1 -> Sum13/1
  x_linearize1/1(y_target) -> Low-Pass Filter/1
  Sum13/1 -> y_linearize2/1(data)
  "Low-Pass Filter "/1 -> des_vel_y/1
  x_target/1 -> " mm to meter "/1
  " mm to meter "/1 -> Sum14/1
  trans_x/1 -> Sum14/2
  Sum14/1 -> x_linearize1/1(data)
  trans_y/1 -> Sum13/2
  Clock5/1 -> z_linearize/2(t)
  z_linearize/1(z_target) -> Sum7/1
  z_target/1 -> " mm to meter"/1
  " mm to meter"/1 -> z_linearize/1(data)
  trans_z/1 -> Sum7/2
  Sum7/1 -> des_vel_z/1

== matlab function controller/yaw_ddelay ==
  data: u input; t input; y output
function y = hold(u, t)
% u: 原始輸入
% t: 當前模擬時間
% y: 輸出，若 t < 1 則為 0，否則輸出 u

if t < 2
    y = 0;
else
    y = u;
end

== matlab function controller/vicon_data1 ==
  data: data input; trans_x output; trans_y output; trans_z output; rot_x output; rot_y output; rot_z output
function [ ...
    trans_x, trans_y, trans_z, rot_x, rot_y, rot_z] = decode_vicon_data(data)
    % Define expected output sizes explicitly
    % Set up each output as an array with dimensions (1x1) or (8x1) as needed.

    % Initialize output arrays

    trans_x = zeros(1, 1, 'double');       % Scalar, double
    trans_y = zeros(1, 1, 'double');       % Scalar, double
    trans_z = zeros(1, 1, 'double');       % Scalar, double
    rot_x = zeros(1, 1, 'double');         % Scalar, double
    rot_y = zeros(1, 1, 'double');         % Scalar, double
    rot_z = zeros(1, 1, 'double');         % Scalar, double

 
    
    % Translation (TransX, TransY, TransZ) - 8 bytes each (double)
    trans_x = typecast(data(33:40), 'double');
    trans_y = typecast(data(41:48), 'double');
    trans_z = typecast(data(49:56), 'double');
    
    % Rotation (RotX, RotY, RotZ) - 8 bytes each (double)
    rot_x = typecast(data(57:64), 'double');
    rot_y = typecast(data(65:72), 'double');
    rot_z = typecast(data(73:80), 'double');
end

== matlab function controller/Subsystem1/y_linearize2 ==
  data: data input; y_target output
function y_target = y_takeoff_smooth(data)
% 延遲 2 秒後開始輸出平滑 takeoff 曲線

    persistent t
    if isempty(t)
        t = 0;
    end

    dt = 0.01;            % 每次呼叫的時間間隔（秒）
    T_delay = 4 ;         % 延遲開始時間（秒）
    T_smooth = 6;        % 平滑上升總時間（秒）
    y_max = data;         % 目標最大高度或位置

    t = t + dt;

    if t < T_delay
        y_target = 0;
    elseif t >= (T_delay + T_smooth)
        y_target = y_max;
    else
        % 將 t 映射到 [0, T_smooth]
        t_s = t - T_delay;
        % 平滑 S 曲線插值
        y_target = y_max * (1 - cos(pi * t_s / T_smooth)) / 2;
    end
end

== matlab function controller/output_data ==
  data: desiredpitch input; desiredroll input; desiredThrottle input; arrayout output; desiredyaw input
% MATLAB Function code
function arrayout  = toarray( desiredpitch,desiredroll,desiredThrottle, desiredyaw )
    % Cast each input value to int32
    desiredroll = single(desiredroll);  
    desiredpitch = single(desiredpitch);  
    desiredyaw = single(desiredyaw);
    desiredThrottle = single(desiredThrottle); 
    
    % Store the values in an array
    arrayout = [desiredroll, desiredpitch, desiredyaw, desiredThrottle];
    
    % Print the values as comma-separated integers with newline
    %fprintf('%d,%d,%d,%d\n', arrayout(1), arrayout(2), arrayout(3), arrayout(4));
end

== matlab function controller/Subsystem1/x_linearize1 ==
  data: data input; y_target output
function y_target = y_takeoff_smooth(data)
% 延遲 2 秒後開始輸出平滑 takeoff 曲線

    persistent t
    if isempty(t)
        t = 0;
    end

    dt = 0.01;            % 每次呼叫的時間間隔（秒）
    T_delay = 4 ;         % 延遲開始時間（秒）
    T_smooth = 6;        % 平滑上升總時間（秒）
    y_max = data;         % 目標最大高度或位置

    t = t + dt;

    if t < T_delay
        y_target = 0;
    elseif t >= (T_delay + T_smooth)
        y_target = y_max;
    else
        % 將 t 映射到 [0, T_smooth]
        t_s = t - T_delay;
        % 平滑 S 曲線插值
        y_target = y_max * (1 - cos(pi * t_s / T_smooth)) / 2;
    end
end

== matlab function controller/Subsystem1/z_linearize ==
  data: data input; z_target output; t input
    function z_target = z_takeoff_smooth(data,t)
    % 平滑 takeoff z_target 輸出：cosine-based interpolation
    
        T = 3;              % 起飛總時間（秒）
        z_max = data;        % 最大高度（公尺）
    
    
        if t >= T
            z_target = z_max;
        else
            % S-curve interpolation：平滑上升
            z_target = z_max * (1 - cos(pi * t / T)) / 2;
        end
    end

== matlab function controller/throttle_out1 ==
  data: velocity_error input; velocity_error output
function velocity_error = scale_error(velocity_error)
%  0–20000 range.

g = 9.81;          % Gravitational acceleration (m/s^2)
m = 0.03;          % Mass of the Crazyflie quadrotor (kg)
Fmax = 1.2;        % Maximum total thrust (N)

K = (m / Fmax) * 20000;   % Scaling factor to map force to the range [0, 20000]

% Convert the velocity error into a scaled thrust command,
% incorporating gravity compensation.
raw_value = (velocity_error  + g) * K;

% Clamp the result within the acceptable thrust command range.
velocity_error = min(max(raw_value, 0), 20000);

end

== matlab function controller/yaw_linearize2 ==
  data: data input; y_target output; t input
function y_target = y_takeoff_smooth(data,t) 
% 延遲 5 秒後平滑起飛，最終輸出最大限制為 10°


    T_delay = 3;          % 延遲開始時間（秒）
    T_smooth = 2;         % 平滑上升總時間（秒）
    y_max_input = data;   % 使用者輸入目標高度或角度
    y_max_limit = 5;     % 最大限制角度（度）
    
    y_max = min(y_max_input, y_max_limit);  % 限制最大值


    if t < T_delay
        y_target = 0;
    elseif t >= (T_delay + T_smooth)
        y_target = y_max;
    else
        % 將 t 映射到 [0, T_smooth]
        t_s = t - T_delay;
        % 平滑 S 曲線插值
        y_target = y_max * (1 - cos(pi * t_s / T_smooth)) / 2;
    end
end

== matlab function controller/input_data1 ==
  data: tran_x input; tran_y input; arrayout output; tran_z input; rot_x input; rot_y input; rot_z input
% MATLAB Function code
function arrayout  = toarray(tran_x, tran_y, tran_z, rot_x, rot_y, rot_z)
    % Cast each input value to int32
    tran_x = single(tran_x);  
    tran_y = single(tran_y);  
    tran_z = single(tran_z);
    rot_x = single(rot_x); 
    rot_y = single(rot_y);
    rot_z = single(rot_z);
    
    % Store the values in an array
    arrayout = [tran_x, tran_y, tran_z, rot_x, rot_y, rot_z];
   
end
